simulink library "hapsrav_library"  (R2017a)
settings: Solver=VariableStepAuto  StartTime=0.0  StopTime=10.0  RelTol=1e-3
values from neighbouring files (symbols this model uses):
  absorb_h = 0:100:40000    [EnergySim.m]
  Adisk = pi * v.R_prop^2    [EnergySim.m]
  alpha_h = absorb_h    [EnergySim.m]
  aoa_data = zeros(n_cl, n)    [EnergySim.m]
  cl_bp = linspace(min_cl, max_cl,n_cl)    [EnergySim.m]
  D = [1       -.0065      288.15          0                   101325 ... (first row only)    [EnergySim.m]    (also in msn_params.m = sqrt((from_x - to_x)^2 + (from_y - to_y)^2); solar_vector.m = time.day + ut_time)
  d2r = pi / 180    (= 0.0174532925199)    [EnergySim.m]    (also in example1.m; example2.m; example3.m; example4.m)
  d_init = sqrt(dx*dx + dy*dy)    [EnergySim.m]    (also in msn_init.m)
  dchi0 = atan2(sin(dchi0), cos(dchi0))    [EnergySim.m]    (also in msn_init.m)
  dT = 0.5    [EnergySim.m]
  dT_fixed = 0.5    [EnergySim.m]
  dT_trig = 30    [EnergySim.m]
  earth_rho = 6378137.0    (= 6378137)    [EnergySim.m]
  fp = solarFP(p.orbit_rho, p.min_axis, p.orbit_dir, ic.x_ctr, ic.y_ctr, sun_az_0)    [EnergySim.m]    (also in load_fp.m = gid_tc(msn_idx).fp; solarFP.m = [1	6	2	nul eul 0	0	0	0	1	0)
  fp_coords = [x_entry y_entry]    [msn_params.m]
  fp_courses = [chi_adj nxt_chi dchi]    [msn_params.m]
  g = 9.80665    [EnergySim.m]
  Gsolar = 1367    [EnergySim.m]
  k = k+1    (= 5)    [EnergySim.m]
  K = D(:,2)    [EnergySim.m]
  lat_init = ic.lat_init_deg * obj.d2r    [EnergySim.m]
  M = time.month    [solar_vector.m]
  max_cl = max(cl_data(:))    [EnergySim.m]
  min_cl = min(cl_data(:))    [EnergySim.m]
  ND2 = load(fullfile(pwd,'nd2_data.mat'))    [EnergySim.m]    (also in nd2_data.mat = [0.0999999999999 0.200000000001 0.3 0.4 0.499999999998 0.700)
  next_init = fp(init_wp, 3)    [EnergySim.m]    (also in msn_init.m)
  pE_init = ic.pE_init    [EnergySim.m]
  pN_init = ic.pN_init    [EnergySim.m]
  r2d = 180 / pi    (= 57.2957795131)    [EnergySim.m]    (also in example1.m; example2.m; example3.m; example4.m)
  rho_SL = 1.225    [EnergySim.m]
  S = 110.4    [EnergySim.m]
  thr_lo_lim = 0.0    (= 0)    [EnergySim.m]
  time_init = struct('year', time.year, 'month', time.month,                  'day', time.day, 'hour', time.hour, 'min', time.min,                  'UTC', time.UTC)    [EnergySim.m]
  to_init = fp(init_wp, 1)    [EnergySim.m]    (also in msn_init.m)
  vgnd_init = sqrt(Vg)    [EnergySim.m]
  vtas_init = veas_init * sqrt(rho_sl/rho_alt)    [EnergySim.m]
  w_alt = 2.0 * w_alt    [EnergySim.m]
  w_xtrack = 2.0 * w_xtrack    [EnergySim.m]
undefined symbols (not defined in the file or in its folder): alpha, alpha_bp, alpha_circ, alt0_rate_init, alt_bp, alt_cmd_mode, alt_init, alt_lim_h, alt_lim_l, alt_rt_lim_periodic, cd_data, charge_eff, chi0_rate_init, chi_cmd_mode, chi_inf, chi_init, cl_data, discharge_eff, DiscIntNeverNeededParam, E_batt_max, E_init, Earth, enableFuzzyLogic, entry_init, epsln, epsln_circ, exit_init, f8_azimuth_offset, fig_eight_time, fp0, fp_coords0, fp_courses0, gamma_lim, hold_time, k_c, K_circ, lat_init_deg, lon_init_deg, max_alpha_bp, max_alt_bp, min_alpha_bp, min_alt_bp, min_axis, motor_eff, mppt_eff, num_motors, orb_dir_init, orb_len_init, orbit_dir, orbit_rho, P_acc, panel_eff, panel_vecs, phi_0, phi_lim, phi_lim_alt, phi_lim_alt_max, phi_lim_alt_min, phi_rt_lim, prop_eff_scale ... (+39)
libraries: simulink x59, hapsrav_library x9, fuzblock x3, atmospheric_library x1, aerolibtransform2 x1
(part 6 of 6)

== matlab function hapsrav_library/hapsrav_main/Kinematic 6DOF/Power Model/sun_position/sun_pos ==
  data: t1 input; sun_az output; t2 input; t3 input; t4 input; t5 input; t6 input; t7 input; l1 input; l2 input; l3 input; sun_zth output; jd output
function [sun_az, sun_zth, jd] = sun_position(t1, t2, t3, t4, t5, t6, t7, l1, l2, l3)
% sun = sun_position(time, location)
%
% This function compute the sun position (zenith and azimuth angle at the observer
% location) as a function of the observer local time and position. 
%
% It is an implementation of the algorithm presented by Reda et Andreas in:
%   Reda, I., Andreas, A. (2003) Solar position algorithm for solar
%   radiation application. National Renewable Energy Laboratory (NREL)
%   Technical report NREL/TP-560-34302. 
% This document is avalaible at www.osti.gov/bridge
%
% This algorithm is based on numerical approximation of the exact equations.
% The authors of the original paper state that this algorithm should be
% precise at +/- 0.0003 degrees. I have compared it to NOAA solar table
% (http://www.srrb.noaa.gov/highlights/sunrise/azel.html) and to USNO solar
% table (http://aa.usno.navy.mil/data/docs/AltAz.html) and found very good
% correspondance (up to the precision of those tables), except for large
% zenith angle, where the refraction by the atmosphere is significant 
% (difference of about 1 degree). Note that in this code the correction 
% for refraction in the atmosphere as been implemented for a temperature 
% of 10C (283 kelvins) and a pressure of 1010 mbar. See the subfunction 
% «sun_topocentric_zenith_angle_calculation» for a possible modification 
% to explicitely model the effect of temperature and pressure as describe
% in Reda & Andreas (2003). 
%
% Input parameters:
%   time: a structure that specify the time when the sun position is
%   calculated. 
%       time.year: year. Valid for [-2000, 6000]
%       time.month: month [1-12]
%       time.day: calendar day [1-31]
%       time.hour: local hour [0-23] (do not use DST)
%       time.min: minute [0-59]
%       time.sec: second [0-59]
%       time.UTC: offset hour from UTC. Local time = Greenwich time + time.UTC
%   This input can also be passed using the Matlab time format ('dd-mmm-yyyy HH:MM:SS'). 
%   In that case, the time has to be specified as UTC time (time.UTC = 0)
%
%   location: a structure that specify the location of the observer
%       location.latitude: latitude (in degrees, north of equator is
%       positive)
%       location.longitude: longitude (in degrees, positive for east of
%       Greenwich)
%       location.altitude: altitude above mean sea level (in meters) 
% 
% Output parameters
%   sun: a structure with the calculated sun position
%       sun.zenith = zenith angle in degrees (angle from the vertical)
%       sun.azimuth = azimuth angle in degrees, eastward from the north. 
% Only the sun zenith and azimuth angles are returned as output, but a lot
% of other parameters are calculated that could also extracted as output of
% this function. 
%
% Exemple of use
%
% location.longitude = -118.592421;
% location.latitude  =   34.181588;
% location.altitude  =  300.0;
% time.year = 2016;
% time.month = 10;
% time.day = 17;  %(do not use DST)
% time.hour = 9;
% time.min =  0;
% time.sec =  0;
% time.UTC = -8;
% 
% sun = sun_position(time, location);
%
% sun = 
% 
%      zenith: 57.8145
%      azimuth: 131.6647
%
% History
%   09/03/2004  Original creation by Vincent Roy (vincent.roy@drdc-rddc.gc.ca)
%   10/03/2004  Fixed a bug in julian_calculation subfunction (was
%               incorrect for year 1582 only), Vincent Roy
%   18/03/2004  Correction to the header (help display) only. No changes to
%               the code. (changed the «elevation» field in «location» structure
%               information to «altitude»), Vincent Roy
%   13/04/2004  Following a suggestion from Jody Klymak (jklymak@ucsd.edu),
%               allowed the 'time' input to be passed as a Matlab time string. 
%   22/08/2005  Following a bug report from Bruce Bowler
%               (bbowler@bigelow.org), modified the julian_calculation function. Bug
%               was 'MATLAB has allowed structure assignment  to a non-empty non-structure 
%               to overwrite the previous value.  This behavior will continue in this release, 
%               but will be an error in a  future version of MATLAB.  For advice on how to 
%               write code that  will both avoid this warning and work in future versions of 
%               MATLAB,  see R14SP2 Release Notes'. Script should now be
%               compliant with futher release of Matlab...

time.year = t1;
time.month = t2;
time.day = t3;
time.hour = t4;
time.min = t5;
time.sec = t6;
time.UTC = t7;

location.longitude = l1;
location.latitude = l2;
location.altitude = l3;

% 1. Calculate the Julian Day, and Century. Julian Ephemeris day, century
% and millenium are calculated using a mean delta_t of 33.184 seconds.  
julian = julian_calculation(time);
jd = mod(julian.day+13, 365.25);

% 2. Calculate the Earth heliocentric longitude, latitude, and radius
% vector (L, B, and R)
earth_heliocentric_position = earth_heliocentric_position_calculation(julian);

% 3. Calculate the geocentric longitude and latitude
sun_geocentric_position = sun_geocentric_position_calculation(earth_heliocentric_position);

% 4. Calculate the nutation in longitude and obliquity (in degrees). 
nutation = nutation_calculation(julian);

% 5. Calculate the true obliquity of the ecliptic (in degrees). 
true_obliquity = true_obliquity_calculation(julian, nutation);

% 6. Calculate the aberration correction (in degrees)
aberration_correction = abberation_correction_calculation(earth_heliocentric_position);

% 7. Calculate the apparent sun longitude in degrees)
apparent_sun_longitude = apparent_sun_longitude_calculation(sun_geocentric_position, nutation, aberration_correction);

% 8. Calculate the apparent sideral time at Greenwich (in degrees)
apparent_stime_at_greenwich = apparent_stime_at_greenwich_calculation(julian, nutation, true_obliquity);

% 9. Calculate the sun right ascension (in degrees)
sun_right_ascension = sun_right_ascension_calculation(apparent_sun_longitude, true_obliquity, sun_geocentric_position);

% 10. Calculate the geocentric sun declination (in degrees). Positive or
% negative if the sun is north or south of the celestial equator. 
sun_geocentric_declination = sun_geocentric_declination_calculation(apparent_sun_longitude, true_obliquity, sun_geocentric_position);

% 11. Calculate the observer local hour angle (in degrees, westward from south).
observer_local_hour = observer_local_hour_calculation(apparent_stime_at_greenwich, location, sun_right_ascension);

% 12. Calculate the topocentric sun position (right ascension, declination and
% right ascension parallax in degrees)
topocentric_sun_position = topocentric_sun_position_calculate(earth_heliocentric_position, location, observer_local_hour, sun_right_ascension, sun_geocentric_declination);

% 13. Calculate the topocentric local hour angle (in degrees)
topocentric_local_hour = topocentric_local_hour_calculate(observer_local_hour, topocentric_sun_position);

% 14. Calculate the topocentric zenith and azimuth angle (in degrees)
sun = sun_topocentric_zenith_angle_calculate(location, topocentric_sun_position, topocentric_local_hour);
sun_az = sun.azimuth;
sun_zth = sun.zenith;
end

%%%%%%%%%%%%%%%%%%%%%%%%%%%
% Subfunction definitions %
%%%%%%%%%%%%%%%%%%%%%%%%%%%

function julian = julian_calculation(t_input)
% This function compute the julian day and julian century from the local
% time and timezone information. Ephemeris are calculated with a delta_t=0
% seconds. 

% If time input is a Matlab time string, extract the information from
% this string and create the structure as defined in the main header of
% this script.
if ~isstruct(t_input)
    tt = datevec(t_input);
    time.UTC=0;
    time.year = tt(1);
    time.month = tt(2);
    time.day = tt(3);
    time.hour = tt(4);
    time.min = tt(5);
    time.sec = tt(6);
else
    time = t_input;
end

if(time.month == 1 || time.month == 2)
    Y = time.year - 1;
    M = time.month + 12;
else
    Y = time.year;
    M = time.month; 
end
ut_time = ((time.hour - time.UTC)/24) + (time.min/(60*24)) + (time.sec/(60*60*24)); % time of day in UT time. 
D = time.day + ut_time; % Day of month in decimal time, ex. 2sd day of month at 12:30:30UT, D=2.521180556

julian = struct('day',0,'ephemeris_day',0,'century',0,'ephemeris_century',0,'ephemeris_millenium',0);

% In 1582, the gregorian calendar was adopted
if(time.year == 1582)
    if(time.month == 10)
        if(time.day <= 4) % The Julian calendar ended on October 4, 1582
            B = 0;    
        elseif(time.day >= 15) % The Gregorian calendar started on October 15, 1582
            A = floor(Y/100);
            B = 2 - A + floor(A/4);    
        else
            disp('This date never existed!. Date automatically set to October 4, 1582');
            time.month = 10;
            time.day = 4; 
            B = 0;
        end
    elseif(time.month<10) % Julian calendar 
        B = 0;
    else % Gregorian calendar
        A = floor(Y/100);
        B = 2 - A + floor(A/4);
    end
    
elseif(time.year<1582) % Julian calendar
    B = 0;
else
    A = floor(Y/100); % Gregorian calendar
    B = 2 - A + floor(A/4);
end

julian.day = floor(365.25*(Y+4716)) + floor(30.6001*(M+1)) + D + B - 1524.5;

delta_t = 0; % 33.184;
julian.ephemeris_day = julian.day + (delta_t/86400);

julian.century = (julian.day - 2451545) / 36525; 

julian.ephemeris_century = (julian.ephemeris_day - 2451545) / 36525;

julian.ephemeris_millenium = julian.ephemeris_century / 10; 
end

function earth_heliocentric_position = earth_heliocentric_position_calculation(julian)
% This function compute the earth position relative to the sun, using
% tabulated values. 

% Tabulated values for the longitude calculation
% L terms  from the original code. 
 L0_terms = [175347046.0 0 0  
 3341656.0 4.6692568 6283.07585  
 34894.0 4.6261 12566.1517  
 3497.0 2.7441 5753.3849  
 3418.0 2.8289 3.5231  
 3136.0 3.6277 77713.7715  
 2676.0 4.4181 7860.4194  
 2343.0 6.1352 3930.2097  
 1324.0 0.7425 11506.7698  
 1273.0 2.0371 529.691  
 1199.0 1.1096 1577.3435  
 990 5.233 5884.927  
 902 2.045 26.298
 857 3.508 398.149  
 780 1.179 5223.694  
 753 2.533 5507.553  
 505 4.583 18849.228  
 492 4.205 775.523  
 357 2.92 0.067  
 317 5.849 11790.629  
 284 1.899 796.298  
 271 0.315 10977.079  
 243 0.345 5486.778  
 206 4.806 2544.314  
 205 1.869 5573.143  
 202 2.4458 6069.777  
 156 0.833 213.299  
 132 3.411 2942.463  
 126 1.083 20.775  
 115 0.645 0.98  
 103 0.636 4694.003  
 102 0.976 15720.839  
 102 4.267 7.114  
 99 6.21 2146.17  
 98 0.68 155.42  
 86 5.98 161000.69  
 85 1.3 6275.96  
 85 3.67 71430.7  
 80 1.81 17260.15  
 79 3.04 12036.46  
 71 1.76 5088.63  
 74 3.5 3154.69  
 74 4.68 801.82  
 70 0.83 9437.76  
 62 3.98 8827.39  
 61 1.82 7084.9  
 57 2.78 6286.6  
 56 4.39 14143.5  
 56 3.47 6279.55  
 52 0.19 12139.55  
 52 1.33 1748.02  
 51 0.28 5856.48  
 49 0.49 1194.45  
 41 5.37 8429.24  
 41 2.4 19651.05  
 39 6.17 10447.39  
 37 6.04 10213.29  
 37 2.57 1059.38  
 36 1.71 2352.87  
 36 1.78 6812.77  
 33 0.59 17789.85  
 30 0.44 83996.85  
 30 2.74 1349.87  
 25 3.16 4690.48];
 
L1_terms = [628331966747.0 0 0  
 206059.0 2.678235 6283.07585  
 4303.0 2.6351 12566.1517  
 425.0 1.59 3.523  
 119.0 5.796 26.298  
 109.0 2.966 1577.344  
 93 2.59 18849.23  
 72 1.14 529.69  
 68 1.87 398.15  
 67 4.41 5507.55  
 59 2.89 5223.69  
 56 2.17 155.42  
 45 0.4 796.3  
 36 0.47 775.52  
 29 2.65 7.11  
 21 5.34 0.98  
 19 1.85 5486.78  
 19 4.97 213.3  
 17 2.99 6275.96  
 16 0.03 2544.31  
 16 1.43 2146.17  
 15 1.21 10977.08
 12 2.83 1748.02  
 12 3.26 5088.63  
 12 5.27 1194.45  
 12 2.08 4694  
 11 0.77 553.57  
 10 1.3 3286.6  
 10 4.24 1349.87  
 9 2.7 242.73  
 9 5.64 951.72  
 8 5.3 2352.87  
 6 2.65 9437.76  
 6 4.67 4690.48]; 
  
L2_terms = [52919.0 0 0  
 8720.0 1.0721 6283.0758  
 309.0 0.867 12566.152  
 27 0.05 3.52  
 16 5.19 26.3  
 16 3.68 155.42  
 10 0.76 18849.23  
 9 2.06 77713.77  
 7 0.83 775.52  
 5 4.66 1577.34  
 4 1.03 7.11  
 4 3.44 5573.14  
 3 5.14 796.3  
 3 6.05 5507.55  
 3 1.19 242.73  
 3 6.12 529.69  
 3 0.31 398.15  
 3 2.28 553.57  
 2 4.38 5223.69  
 2 3.75 0.98];

L3_terms =[289.0 5.844 6283.076  
 35 0 0  
 17 5.49 12566.15  
 3 5.2 155.42  
 1 4.72 3.52  
 1 5.3 18849.23  
 1 5.97 242.73]; 
 
L4_terms = [114.0 3.142 0  
 8 4.13 6283.08  
 1 3.84 12566.15];

L5_terms = [1 3.14 0]; 

A0 = L0_terms(:,1);
B0 = L0_terms(:,2);
C0 = L0_terms(:,3);

A1 = L1_terms(:,1);
B1 = L1_terms(:,2);
C1 = L1_terms(:,3);

A2 = L2_terms(:,1);
B2 = L2_terms(:,2);
C2 = L2_terms(:,3);

A3 = L3_terms(:,1);
B3 = L3_terms(:,2);
C3 = L3_terms(:,3);

A4 = L4_terms(:,1);
B4 = L4_terms(:,2);
C4 = L4_terms(:,3);

A5 = L5_terms(:,1);
B5 = L5_terms(:,2);
C5 = L5_terms(:,3);

JME = julian.ephemeris_millenium;

% Compute the Earth Heliocentric longitude from the tabulated values. 
L0 = sum(A0 .* cos(B0 + (C0 * JME)));
L1 = sum(A1 .* cos(B1 + (C1 * JME)));
L2 = sum(A2 .* cos(B2 + (C2 * JME)));
L3 = sum(A3 .* cos(B3 + (C3 * JME)));
L4 = sum(A4 .* cos(B4 + (C4 * JME)));
L5 = A5 .* cos(B5 + (C5 * JME));


earth_heliocentric_position = struct('longitude',0,'latitude',0,'radius',0);

earth_heliocentric_position.longitude = (L0 + (L1 * JME) + (L2 * JME^2) + (L3 * JME^3) + (L4 * JME^4) + (L5 * JME^5)) / 1e8; 
% Convert the longitude to degrees. 
earth_heliocentric_position.longitude = earth_heliocentric_position.longitude * 180/pi;
% Limit the range to [0,360[;
earth_heliocentric_position.longitude = set_to_range(earth_heliocentric_position.longitude, 0, 360);

% Tabulated values for the earth heliocentric latitude. 
% B terms  from the original code. 
 B0_terms = [280.0 3.199 84334.662  
 102.0 5.422 5507.553  
 80 3.88 5223.69  
 44 3.7 2352.87  
 32 4 1577.34]; 
  
B1_terms = [9 3.9 5507.55  
 6 1.73 5223.69]; 

A0 = B0_terms(:,1);
B0 = B0_terms(:,2);
C0 = B0_terms(:,3);

A1 = B1_terms(:,1);
B1 = B1_terms(:,2);
C1 = B1_terms(:,3);

L0 = sum(A0 .* cos(B0 + (C0 * JME)));
L1 = sum(A1 .* cos(B1 + (C1 * JME)));

earth_heliocentric_position.latitude = (L0 + (L1 * JME)) / 1e8; 
% Convert the latitude to degrees. 
earth_heliocentric_position.latitude = earth_heliocentric_position.latitude * 180/pi;
% Limit the range to [0,360];
earth_heliocentric_position.latitude = set_to_range(earth_heliocentric_position.latitude, 0, 360);

% Tabulated values for radius vector. 
% R terms from the original code
R0_terms = [ 100013989.0 0 0  
 1670700.0 3.0984635 6283.07585  
 13956.0 3.05525 12566.1517   
 3084.0 5.1985 77713.7715  
 1628.0 1.1739 5753.3849  
 1576.0 2.8469 7860.4194  
 925.0 5.453 11506.77  
 542.0 4.564 3930.21  
 472.0 3.661 5884.927  
 346.0 0.964 5507.553  
 329.0 5.9 5223.694  
 307.0 0.299 5573.143  
 243.0 4.273 11790.629  
 212.0 5.847 1577.344  
 186.0 5.022 10977.079  
 175.0 3.012 18849.228  
 110.0 5.055 5486.778  
 98 0.89 6069.78  
 86 5.69 15720.84  
 86 1.27 161000.69  
 85 0.27 17260.15  
 63 0.92 529.69  
 57 2.01 83996.85  
 56 5.24 71430.7  
 49 3.25 2544.31  
 47 2.58 775.52  
 45 5.54 9437.76  
 43 6.01 6275.96  
 39 5.36 4694  
 38 2.39 8827.39  
 37 0.83 19651.05  
 37 4.9 12139.55  
 36 1.67 12036.46  
 35 1.84 2942.46  
 33 0.24 7084.9  
 32 0.18 5088.63  
 32 1.78 398.15  
 28 1.21 6286.6  
 28 1.9 6279.55  
 26 4.59 10447.39];
   
R1_terms = [ 103019.0 1.10749 6283.07585  
 1721.0 1.0644 12566.1517  
 702.0 3.142 0  
 32 1.02 18849.23  
 31 2.84 5507.55  
 25 1.32 5223.69  
 18 1.42 1577.34  
 10 5.91 10977.08  
 9 1.42 6275.96  
 9 0.27 5486.78];
  
R2_terms = [4359.0 5.7846 6283.0758  
 124.0 5.579 12566.152  
 12 3.14 0  
 9 3.63 77713.77  
 6 1.87 5573.14  
 3 5.47 18849];
 
R3_terms = [145.0 4.273 6283.076  
 7 3.92 12566.15];

R4_terms = [4 2.56 6283.08];


A0 = R0_terms(:,1);
B0 = R0_terms(:,2);
C0 = R0_terms(:,3);

A1 = R1_terms(:,1);
B1 = R1_terms(:,2);
C1 = R1_terms(:,3);

A2 = R2_terms(:,1);
B2 = R2_terms(:,2);
C2 = R2_terms(:,3);

A3 = R3_terms(:,1);
B3 = R3_terms(:,2);
C3 = R3_terms(:,3);

A4 = R4_terms(:,1);
B4 = R4_terms(:,2);
C4 = R4_terms(:,3);

% Compute the Earth heliocentric radius vector
L0 = sum(A0 .* cos(B0 + (C0 * JME)));
L1 = sum(A1 .* cos(B1 + (C1 * JME)));
L2 = sum(A2 .* cos(B2 + (C2 * JME)));
L3 = sum(A3 .* cos(B3 + (C3 * JME)));
L4 = A4 .* cos(B4 + (C4 * JME));

% Units are in AU
earth_heliocentric_position.radius = (L0 + (L1 * JME) + (L2 * JME^2) + (L3 * JME^3) + (L4 * JME^4)) / 1e8; 

end

function sun_geocentric_position = sun_geocentric_position_calculation(earth_heliocentric_position)
% This function compute the sun position relative to the earth. 
sun_geocentric_position = struct('longitude',0,'latitude',0);

sun_geocentric_position.longitude = earth_heliocentric_position.longitude + 180;
% Limit the range to [0,360];
sun_geocentric_position.longitude = set_to_range(sun_geocentric_position.longitude, 0, 360);

sun_geocentric_position.latitude = -earth_heliocentric_position.latitude;
% Limit the range to [0,360]
sun_geocentric_position.latitude = set_to_range(sun_geocentric_position.latitude, 0, 360);
end

function nutation = nutation_calculation(julian)
% This function compute the nutation in longtitude and in obliquity, in
% degrees. 

% All Xi are in degrees. 
JCE = julian.ephemeris_century;

% 1. Mean elongation of the moon from the sun 
p = [(1/189474) -0.0019142 445267.11148 297.85036];
% X0 = polyval(p, JCE);
X0 = p(1) * JCE^3 + p(2) * JCE^2 + p(3) * JCE + p(4); % This is faster than polyval...

% 2. Mean anomaly of the sun (earth)
p = [-(1/300000) -0.0001603 35999.05034 357.52772];
% X1 = polyval(p, JCE);
X1 = p(1) * JCE^3 + p(2) * JCE^2 + p(3) * JCE + p(4); 

% 3. Mean anomaly of the moon
p = [(1/56250) 0.0086972 477198.867398 134.96298];
% X2 = polyval(p, JCE);
X2 = p(1) * JCE^3 + p(2) * JCE^2 + p(3) * JCE + p(4); 

% 4. Moon argument of latitude
p = [(1/327270) -0.0036825 483202.017538 93.27191];
% X3 = polyval(p, JCE);
X3 = p(1) * JCE^3 + p(2) * JCE^2 + p(3) * JCE + p(4); 

% 5. Longitude of the ascending node of the moon's mean orbit on the
% ecliptic, measured from the mean equinox of the date
p = [(1/450000) 0.0020708 -1934.136261 125.04452];
% X4 = polyval(p, JCE);
X4 = p(1) * JCE^3 + p(2) * JCE^2 + p(3) * JCE + p(4); 

% Y tabulated terms from the original code
Y_terms =  [0 0 0 0 1  
 -2 0 0 2 2  
 0 0 0 2 2  
 0 0 0 0 2  
 0 1 0 0 0  
 0 0 1 0 0  
 -2 1 0 2 2  
 0 0 0 2 1  
 0 0 1 2 2  
 -2 -1 0 2 2  
 -2 0 1 0 0  
 -2 0 0 2 1  
 0 0 -1 2 2  
 2 0 0 0 0  
 0 0 1 0 1  
 2 0 -1 2 2  
 0 0 -1 0 1  
 0 0 1 2 1  
 -2 0 2 0 0  
 0 0 -2 2 1  
 2 0 0 2 2  
 0 0 2 2 2  
 0 0 2 0 0  
 -2 0 1 2 2  
 0 0 0 2 0  
 -2 0 0 2 0  
 0 0 -1 2 1  
 0 2 0 0 0  
 2 0 -1 0 1  
 -2 2 0 2 2  
 0 1 0 0 1  
 -2 0 1 0 1  
 0 -1 0 0 1  
 0 0 2 -2 0  
 2 0 -1 2 1  
 2 0 1 2 2  
 0 1 0 2 2  
 -2 1 1 0 0  
 0 -1 0 2 2  
 2 0 0 2 1  
 2 0 1 0 0  
 -2 0 2 2 2  
 -2 0 1 2 1  
 2 0 -2 0 1  
 2 0 0 0 1  
 0 -1 1 0 0  
 -2 -1 0 2 1  
 -2 0 0 0 1  
 0 0 2 2 1  
 -2 0 2 0 1  
 -2 1 0 2 1  
 0 0 1 -2 0  
 -1 0 1 0 0  
 -2 1 0 0 0  
 1 0 0 0 0  
 0 0 1 2 0  
 0 0 -2 2 2  
 -1 -1 1 0 0  
 0 1 1 0 0  
 0 -1 1 2 2  
 2 -1 -1 2 2  
 0 0 3 2 2  
 2 -1 0 2 2];

nutation_terms = [ -171996 -174.2 92025 8.9  
 -13187 -1.6 5736 -3.1  
 -2274 -0.2 977 -0.5  
 2062 0.2 -895 0.5  
 1426 -3.4 54 -0.1  
 712 0.1 -7 0  
 -517 1.2 224 -0.6  
 -386 -0.4 200 0  
 -301 0 129 -0.1  
 217 -0.5 -95 0.3  
 -158 0 0 0  
 129 0.1 -70 0  
 123 0 -53 0  
 63 0 0 0  
 63 0.1 -33 0  
 -59 0 26 0  
 -58 -0.1 32 0  
 -51 0 27 0  
 48 0 0 0  
 46 0 -24 0  
 -38 0 16 0  
 -31 0 13 0  
 29 0 0 0  
 29 0 -12 0  
 26 0 0 0  
 -22 0 0 0  
 21 0 -10 0  
 17 -0.1 0 0  
 16 0 -8 0  
 -16 0.1 7 0  
 -15 0 9 0  
 -13 0 7 0  
 -12 0 6 0  
 11 0 0 0  
 -10 0 5 0  
 -8 0 3 0  
 7 0 -3 0  
 -7 0 0 0  
 -7 0 3 0  
 -7 0 3 0  
 6 0 0 0  
 6 0 -3 0  
 6 0 -3 0  
 -6 0 3 0  
 -6 0 3 0  
 5 0 0 0  
 -5 0 3 0  
 -5 0 3 0  
 -5 0 3 0  
 4 0 0 0  
 4 0 0 0  
 4 0 0 0  
 -4 0 0 0  
 -4 0 0 0  
 -4 0 0 0  
 3 0 0 0  
 -3 0 0 0  
 -3 0 0 0  
 -3 0 0 0  
 -3 0 0 0  
 -3 0 0 0  
 -3 0 0 0  
 -3 0 0 0];

% Using the tabulated values, compute the delta_longitude and
% delta_obliquity. 
Xi = [X0
    X1
    X2
    X3
    X4];

tabulated_argument = (Y_terms * Xi) * pi/180;

delta_longitude = ((nutation_terms(:,1) + (nutation_terms(:,2) * JCE))) .* sin(tabulated_argument);
delta_obliquity = ((nutation_terms(:,3) + (nutation_terms(:,4) * JCE))) .* cos(tabulated_argument);

% Nutation in longitude
nutation.longitude = sum(delta_longitude) / 36000000;

% Nutation in obliquity
nutation.obliquity = sum(delta_obliquity) / 36000000;
end

function true_obliquity = true_obliquity_calculation(julian, nutation)
% This function compute the true obliquity of the ecliptic. 


p = [2.45 5.79 27.87 7.12 -39.05 -249.67 -51.38 1999.25 -1.55 -4680.93 84381.448];
% mean_obliquity = polyval(p, julian.ephemeris_millenium/10);

U = julian.ephemeris_millenium/10;
mean_obliquity = p(1)*U^10 + p(2)*U^9 + p(3)*U^8 + p(4)*U^7 + p(5)*U^6 + p(6)*U^5 + p(7)*U^4 + p(8)*U^3 + p(9)*U^2 + p(10)*U + p(11);


true_obliquity = (mean_obliquity/3600) + nutation.obliquity;
end

function aberration_correction = abberation_correction_calculation(earth_heliocentric_position)
% This function compute the aberration_correction, as a function of the
% earth-sun distance. 

aberration_correction = -20.4898/(3600*earth_heliocentric_position.radius);
end

function apparent_sun_longitude = apparent_sun_longitude_calculation(sun_geocentric_position, nutation, aberration_correction)
% This function compute the sun apparent longitude

apparent_sun_longitude = sun_geocentric_position.longitude + nutation.longitude + aberration_correction;
end

function apparent_stime_at_greenwich = apparent_stime_at_greenwich_calculation(julian, nutation, true_obliquity)
% This function compute the apparent sideral time at Greenwich. 

JD = julian.day;
JC = julian.century;

% Mean sideral time, in degrees
mean_stime = 280.46061837 + (360.98564736629*(JD-2451545)) + (0.000387933*JC^2) - (JC^3/38710000);

% Limit the range to [0-360];
mean_stime = set_to_range(mean_stime, 0, 360);

apparent_stime_at_greenwich = mean_stime + (nutation.longitude * cos(true_obliquity * pi/180));
end

function sun_right_ascension = sun_right_ascension_calculation(apparent_sun_longitude, true_obliquity, sun_geocentric_position)
% This function compute the sun right ascension. 

argument_numerator = (sin(apparent_sun_longitude * pi/180) * cos(true_obliquity * pi/180)) - ...
    (tan(sun_geocentric_position.latitude * pi/180) * sin(true_obliquity * pi/180));
argument_denominator = cos(apparent_sun_longitude * pi/180);

sun_right_ascension = atan2(argument_numerator, argument_denominator) * 180/pi;
% Limit the range to [0,360];
sun_right_ascension = set_to_range(sun_right_ascension, 0, 360);
end

function sun_geocentric_declination = sun_geocentric_declination_calculation(apparent_sun_longitude, true_obliquity, sun_geocentric_position)

argument = (sin(sun_geocentric_position.latitude * pi/180) * cos(true_obliquity * pi/180)) + ...
    (cos(sun_geocentric_position.latitude * pi/180) * sin(true_obliquity * pi/180) * sin(apparent_sun_longitude * pi/180));

sun_geocentric_declination = asin(argument) * 180/pi;
end

function observer_local_hour = observer_local_hour_calculation(apparent_stime_at_greenwich, location, sun_right_ascension)

observer_local_hour = apparent_stime_at_greenwich + location.longitude - sun_right_ascension;
% Set the range to [0-360]
observer_local_hour = set_to_range(observer_local_hour, 0, 360);

end

function topocentric_sun_position = topocentric_sun_position_calculate(earth_heliocentric_position, location, observer_local_hour, sun_right_ascension, sun_geocentric_declination)
% This function compute the sun position (right ascension and declination)
% with respect to the observer local position at the Earth surface. 

% Equatorial horizontal parallax of the sun in degrees
eq_horizontal_parallax = 8.794 / (3600 * earth_heliocentric_position.radius);

% Term u, used in the following calculations (in radians)
u = atan(0.99664719 * tan(location.latitude * pi/180));

% Term x, used in the following calculations
x = cos(u) + ((location.altitude/6378140) * cos(location.latitude * pi/180));

% Term y, used in the following calculations
y = (0.99664719 * sin(u)) + ((location.altitude/6378140) * sin(location.latitude * pi/180));

% Parallax in the sun right ascension (in radians)
nominator = -x * sin(eq_horizontal_parallax * pi/180) * sin(observer_local_hour * pi/180);
denominator = cos(sun_geocentric_declination * pi/180) - (x * sin(eq_horizontal_parallax * pi/180) * cos(observer_local_hour * pi/180));
sun_right_ascension_parallax = atan2(nominator, denominator);
% Conversion to degrees. 
topocentric_sun_position.right_ascension_parallax = sun_right_ascension_parallax * 180/pi;

% Topocentric sun right ascension (in degrees)
topocentric_sun_position.right_ascension = sun_right_ascension + (sun_right_ascension_parallax * 180/pi);

% Topocentric sun declination (in degrees)
nominator = (sin(sun_geocentric_declination * pi/180) - (y*sin(eq_horizontal_parallax * pi/180))) * cos(sun_right_ascension_parallax);
denominator = cos(sun_geocentric_declination * pi/180) - (x*sin(eq_horizontal_parallax * pi/180)) * cos(observer_local_hour * pi/180);
topocentric_sun_position.declination = atan2(nominator, denominator) * 180/pi;
end

function topocentric_local_hour = topocentric_local_hour_calculate(observer_local_hour, topocentric_sun_position)
% This function compute the topocentric local jour angle in degrees

topocentric_local_hour = observer_local_hour - topocentric_sun_position.right_ascension_parallax;
end

function sun = sun_topocentric_zenith_angle_calculate(location, topocentric_sun_position, topocentric_local_hour)
% This function compute the sun zenith angle, taking into account the
% atmospheric refraction. A default temperature of 283K and a
% default pressure of 1010 mbar are used. 

% Topocentric elevation, without atmospheric refraction
argument = (sin(location.latitude * pi/180) * sin(topocentric_sun_position.declination * pi/180)) + ...
    (cos(location.latitude * pi/180) * cos(topocentric_sun_position.declination * pi/180) * cos(topocentric_local_hour * pi/180));
true_elevation = asin(argument) * 180/pi;

% Atmospheric refraction correction (in degrees)
argument = true_elevation + (10.3/(true_elevation + 5.11));
refraction_corr = 1.02 / (60 * tan(argument * pi/180));

% For exact pressure and temperature correction, use this, 
% with P the pressure in mbar amd T the temperature in Kelvins:
% refraction_corr = (P/1010) * (283/T) * 1.02 / (60 * tan(argument * pi/180));

% Apparent elevation
if(true_elevation > -5)
    apparent_elevation = true_elevation + refraction_corr;
else
    apparent_elevation = true_elevation;
end

sun.zenith = 90 - apparent_elevation;


% Topocentric azimuth angle. The +180 conversion is to pass from astronomer
% notation (westward from south) to navigation notation (eastward from
% north);
nominator = sin(topocentric_local_hour * pi/180);
denominator = (cos(topocentric_local_hour * pi/180) * sin(location.latitude * pi/180)) - ...
    (tan(topocentric_sun_position.declination * pi/180) * cos(location.latitude * pi/180));
sun.azimuth = (atan2(nominator, denominator) * 180/pi) + 180;
% Set the range to [0-360]
sun.azimuth = set_to_range(sun.azimuth, 0, 360);
end

function var = set_to_range(var, min_interval, max_interval)
% if(var>0)
%     var = var - max_interval * floor(var/max_interval);
% else
%     var = var - max_interval * ceil(var/max_interval);
% end
% 
% if(var<min_interval)
%     var = var + max_interval;
% end

var = var - max_interval * floor(var/max_interval);

if(var<min_interval)
    var = var + max_interval;
end
end

== matlab function hapsrav_library/hapsrav_main/Kinematic 6DOF/Power Model/sun_position/time_update ==
  data: time_init input; t_new output; sim_secs input
function t_new = fcn(time_init, sim_secs)
coder.extrinsic('datetime');
coder.extrinsic('datevec');

time_now = time_init + sim_secs;
t_new = zeros(6,1);

    if ~coder.target('MATLAB')
        coder.cinclude('<stdio.h>');
        coder.cinclude('<time.h>');
        coder.cinclude('date_vec.h');

        t_new(1) = coder.ceval('get_year',time_now);
        t_new(2) = coder.ceval('get_month',time_now);
        t_new(3) = coder.ceval('get_day',time_now);
        t_new(4) = coder.ceval('get_hour',time_now);
        t_new(5) = coder.ceval('get_min',time_now);
        t_new(6) = coder.ceval('get_sec',time_now);
    else
        dt_now = datetime(time_now,'ConvertFrom','posixtime');
        t_new_tmp = datevec(dt_now);
        t_new = t_new_tmp';
    end
end

== matlab function hapsrav_library/Cmd - Parametric/Chi Cmd/Circular Vector Fields/MATLAB Function1 ==
  data: av_x input; av_y input; d output; x_c input; y_c input; orbit_dir input; g output; beta output; r_c input; chi_d output; k_c input
function [d,g,beta,chi_d] = relPosn(av_x, av_y, x_c, y_c, orbit_dir, r_c, k_c)

x = av_x;
y = av_y;
% x_c = to_x
% y_c = to_y;

dx = x - x_c;
dy = y - y_c;

d = sqrt(dx * dx + dy * dy);
g = atan2(dy, dx);       % correct as dy, dx

ang_y = k_c * (d - r_c);
ang_x = r_c;

if (orbit_dir)
    % CCW
    chi_d = g - pi/2 - atan(ang_y/ ang_x);
else
    % CW
    chi_d = g + pi/2 + atan(ang_y/ ang_x);
end

chi_d = wrap2pi(chi_d);

% Compute beta
d_err = d - r_c;
k_r = k_c / r_c;
beta = k_r / (1 + (k_r * d_err)^2);


end

function wrpd = wrap2pi(angl)

% Wrap to +/- pi
if (angl > pi)
    wrpd = -pi + (angl - pi);
elseif (angl < -pi)
    wrpd = 2 * pi + angl;
else
    wrpd = angl;
end

end

== matlab function hapsrav_library/hapsrav_main/Kinematic 6DOF/Selectable Modes/Trajectory_Optimization/Roll/roll_angle/Limited Integration ==
  data: u input; y0 output; T input; uplim input; lolim input; x0 input; x1 output
function [y0,x1] = lim_integr(u, T, uplim, lolim, x0)

K = 1.0;

y0   = x0 + K * T/2 * u;
y0 = max(min(y0, uplim), lolim);
x1   = y0 + K * T/2 * u;

end

== matlab function hapsrav_library/Cmd - Parametric/Chi Cmd/Circular Vector Fields/MATLAB Function3 ==
  data: chi input; chi_cmd output; d input; g input; chi_d input; beta input; Vg input; alpha input; e input; K input
function chi_cmd = chiCmdCirc(chi, d, g, chi_d, beta, Vg, alpha, e, K)

chi_err = wrap2pi(chi - chi_d);
angl = chi - g;
angl = wrap2pi(angl);

chi_cmd = chi + Vg * sin(angl) / alpha / d;
chi_cmd = chi_cmd - beta * Vg * cos(angl) / alpha;

satVal = sat_val(chi_err, e);
chi_cmd = chi_cmd - K * satVal / alpha;
chi_cmd = wrap2pi(chi_cmd);

end

function satVal = sat_val(u,epsln)

x = u / epsln;

if (abs(x) <= 1)
    satVal = x;
else
    satVal = sign(x);
end

end

function wrpd = wrap2pi(angl)

% Wrap to +/- pi
if (angl > pi)
    wrpd = -pi + (angl - pi);
elseif (angl < -pi)
    wrpd = 2 * pi + angl;
else
    wrpd = angl;
end

end

== matlab function hapsrav_library/hapsrav_main/Kinematic 6DOF/Selectable Modes/Waypoint_Navigation/Course/MATLAB Function2 ==
  data: ref input; circ_err output; posn input
function circ_err  = circErr(ref, posn)
% Assumes that both angles are limited to the range +/-pi
% Replace this function with a summing junction
% to see why it's needed.  Go thru a sign change
% in the error.

s1 = sign(ref);
s2 = sign(posn);

err = ref - posn;

if (s1 > s2),
    if (abs(err) > pi),
        err = err - 2*pi;
    end
elseif (s2 > s1),
    if (abs(err) > pi),
        err = 2*pi + err;
    end
end

% When error is exactly +/-pi, want to add option to continue
% turning along same direction
circ_err = err;

end

== matlab function hapsrav_library/hapsrav_main/Kinematic 6DOF/Selectable Modes/Waypoint_Navigation/Course/chi_dot/Limited Integration ==
  data: u input; y0 output; T input; lim input; x0 input; x1 output
function [y0,x1] = lim_integr(u, T, lim, x0)

K = 1.0;

y0   = x0 + K * T/2 * u;

y0 = max(min(y0, lim), -lim);

x1   = y0 + K * T/2 * u;

end

== stateflow chart hapsrav_library/Cmd - Parametric/Chi Cmd/Flight Plan/Mission Director/Fly Away Detection ==
  state Not_Fly_Away
    %
    entry:
    fly_away_flg = false;
  state Counting
    %
    entry:
    fly_away_ctr = 500;
    during:
    fly_away_ctr = fly_away_ctr - 1;
  state Fly_Away
    %
    entry:
    fly_away_flg = true;
  (default) -> Not_Fly_Away
  Fly_Away -> Not_Fly_Away : [d2n >= turn_rad]
  Counting -> Not_Fly_Away [order 1] : [~retreating]
  Not_Fly_Away -> Counting : [(d2n < turn_rad) && ...
      | retreating]
  Counting -> Fly_Away [order 2] : [fly_away_ctr == 0]
  data: d2n input; retreating input; turn_rad input; fly_away_flg output boolean; fly_away_ctr local

== matlab function hapsrav_library/Cmd - Parametric/Chi Cmd/Flight Plan/Mission Director/MATLAB Function ==
  data: wp_upd input; wp_upd_old input; wp_to output; wp_entry input; wp_curr input; wp_next input
function wp_to  = fcn(wp_upd, wp_upd_old, wp_entry, wp_curr, wp_next)

if (wp_upd == 0)
    wp_to = wp_entry;
elseif (wp_upd ~= wp_upd_old)
    wp_to = wp_next;
else
    wp_to = wp_curr;
end

end

== stateflow chart hapsrav_library/Cmd - Parametric/Chi Cmd/Flight Plan/Mission Director/Mission Director ==
  state Not_Entry_Mode
    state Orbit_Holding_Mode
      state Pattern_Hold_Entry
        %
        entry:
        orbit_timer = 50 * orbit_time;
        sweeping = false;
        state_flg = -2;
      state Pattern_Hold
        state Entry
          %
          entry:
          nav_mode = 3;
          state_flg = -3;
        state Sweep_Exit_Mode
          entry:
          sweeping = true;
          state_flg = 5;
        state Timer_Exit_Mode
          entry:
          state_flg = 4;
          during:
          orbit_timer = orbit_timer - 1;
        (default) -> Not_Entry_Mode.Orbit_Holding_Mode.Pattern_Hold.Entry
        Not_Entry_Mode.Orbit_Holding_Mode.Pattern_Hold.Entry -> Sweep_Exit_Mode [order 2] : [sweep_flg]
        Not_Entry_Mode.Orbit_Holding_Mode.Pattern_Hold.Entry -> Timer_Exit_Mode [order 1] : [~sweep_flg]
      state Fly_Over_Mode	% 2
        %
        entry:
        if (nav_mode ~= 0)
        nav_mode = 2;
        end
        delay_timer = 50 * 4;
        state_flg = 3;
        during:
        delay_timer = delay_timer -1;
      (default) -> Pattern_Hold_Entry
      Pattern_Hold_Entry -> Pattern_Hold [order 1] : [fly_over_flg ~= 2]
      Pattern_Hold_Entry -> Fly_Over_Mode	% 2 [order 2] : [fly_over_flg == 2]
      Fly_Over_Mode	% 2 -> Pattern_Hold : [delay_timer == 0]
    state Entry
      entry:
      state_flg = -1;
    state Path_Following_Mode		% 2
      %
      entry:
      nav_mode = 2;
      state_flg = 2;
    state Turning_Mode 	% 0
      %
      entry:
      nav_mode = 1;
      state_flg = 1;
    (default) -> Not_Entry_Mode.Entry
    Not_Entry_Mode.Entry -> Orbit_Holding_Mode [order 1] : [orbit_flg]
    Not_Entry_Mode.Entry -> Turning_Mode 	% 0 [order 2] : [~orbit_flg]
        | {wp_upd = wp_upd + 1;}
    Orbit_Holding_Mode -> (junction 183) [order 2] : [~sweep_flg && sweeping]
    Orbit_Holding_Mode -> (junction 183) [order 1] : [orbit_timer == 0]
    Path_Following_Mode		% 2 -> Orbit_Holding_Mode [order 2] : [orbit_flg && ...
        | (d2n < prox_dist)]
    (junction 183) -> Path_Following_Mode		% 2 : {wp_upd = wp_upd + 1;}
    Path_Following_Mode		% 2 -> Turning_Mode 	% 0 [order 1] : [~orbit_flg && ...
        | ((d2n < prox_dist) || fly_away_flg)]
        | {wp_upd = wp_upd + 1;}
    Turning_Mode 	% 0 -> Path_Following_Mode		% 2 : [d2n >= prox_dist]
  state Entry_Mode	% 1
    %
    entry:
    wp_upd = 0;
    msn_rst = 1;
    nav_mode = 0;
    state_flg = 0;
    %
    during:
    msn_rst = 0;
  (default) -> Entry_Mode	% 1
  Entry_Mode	% 1 -> Not_Entry_Mode : [d2n < prox_dist]
  Not_Entry_Mode -> Entry_Mode	% 1 : % 2
      | [Ovrd]
  data: Ovrd input; d2n input; wp_upd output; nav_mode output; prox_dist input; orbit_time input; msn_rst output; orbit_timer local; delay_timer local; orbit_flg input; fly_over_flg input; fly_away_flg input; sweep_flg input; sweeping local boolean; state_flg output

== matlab function hapsrav_library/Cmd - Parametric/Chi Cmd/Flight Plan/Mission Director/Nav Leg/Flight Plan/Realtime FP/MATLAB Function ==
  data: fp output; fp_courses output; fp_coords output; maj_axis input; min_axis input; orbit_dir input; x_ctr input; y_ctr input; az input
function [fp, fp_courses, fp_coords] = update_fp(maj_axis, min_axis, orbit_dir, x_ctr, y_ctr, az)

nc = x_ctr;
ec = y_ctr;

rho = min_axis;
drho = maj_axis - min_axis;

nu_ctr = nc + drho * cos(az);
eu_ctr = ec + drho * sin(az);

nur = nu_ctr - rho * sin(az);
eur = eu_ctr + rho * cos(az);
nul = nu_ctr + rho * sin(az);
eul = eu_ctr - rho * cos(az);

nl_ctr = nc - drho * cos(az);
el_ctr = ec - drho * sin(az);

nlr = nl_ctr - rho * sin(az);
elr = el_ctr + rho * cos(az);
nll = nl_ctr + rho * sin(az);
ell = el_ctr - rho * cos(az);

% orbit direction: 1 - CCW, 0 - CW
if (orbit_dir)  % CCW
    fp = [1	6	2	nur eur 0	0	0	0	1	0;
        2	1	3   nu_ctr eu_ctr 1	min_axis	1	180	3	5;
        3	2	4   nul eul 0	0	0	0	1	0;
        4	3	5   nll ell 0	0	0	0	1	0;
        5	4	6   nl_ctr el_ctr 1	min_axis	1	180	3	5;
        6	5	1   nlr elr 0	0	0	0	1	0];
else    % CW
    fp = [1	6	2	nul eul 0	0	0	0	1	0;
        2	1	3	nu_ctr eu_ctr 1	min_axis	0	180	3	5;
        3	2	4	nur eur 0	0	0	0	1	0;
        4	3	5	nlr elr 0	0	0	0	1	0;
        5	4	6	nl_ctr el_ctr 1	min_axis	0	180	3	5;
        6	5	1	nll ell 0	0	0	0	1	0];
end

[fp_courses, fp_coords] = msn_params(fp);

end

function [fp_courses, fp_coords] = msn_params(fp)
%
num_wp = 6;

chi_nom    = zeros(num_wp,1);	% course of this leg (to, from)
chi_adj    = zeros(num_wp,1);   % course of next leg (next, to)
nxt_chi    = zeros(num_wp,1);   % course of next leg (next, to)
dchi       = zeros(num_wp,1);   % change in course

x_entry = zeros(num_wp,1);
y_entry = zeros(num_wp,1);

for i = 1:num_wp
    
    % Compute chi, next_chi, delta_chi
    to_wp = fp(i, 1);
    from_wp = fp(i, 2);
    
    to_x = fp(to_wp, 4);
    to_y = fp(to_wp, 5);
    from_x = fp(from_wp, 4);
    from_y = fp(from_wp, 5);
    
    dy = to_y - from_y;
    dx = to_x - from_x;
    chi_nom(i) = atan2(dy,dx);
    
    % Compute entry point for intercept patternholds
    % whenever intercept and orbit are both defined
    if (fp(i,10) == 3)
%         % Circle parameters
%         %rho = fp(to_wp, 7);
%         %D = sqrt((from_x - to_x)^2 + (from_y - to_y)^2);
%         %gamma = pi/2 - acos(rho / D);
%         gamma = pi/2;
%         %De = sqrt(D*D - rho*rho);
%         De = 0.0;
%         
%         if (fp(to_wp,8) > 0)    % CCW
%             chi_adj(i) = chi_nom(i) + gamma;
%         else                    % CW
%             chi_adj(i) = chi_nom(i) - gamma;
%         end
%         
%         %y_entry(i) = from_y + De * sin(chi_adj(i));
%         %x_entry(i) = from_x + De * cos(chi_adj(i));
%         
%         y_entry(i) = from_y;
%         x_entry(i) = from_x;

        % Circle parameters
        rho = fp(to_wp, 7);
        D = sqrt((from_x - to_x)^2 + (from_y - to_y)^2);
        % problem when rho > D
        if (rho > D)
            gamma = pi/2;
            De = 0.0;
        else 
            gamma = pi/2 - acos(rho / D);
            De = sqrt(D*D - rho*rho);
        end
        
        if (fp(to_wp,8) > 0)    % CCW
            chi_adj(i) = chi_nom(i) + gamma;
        else                    % CW
            chi_adj(i) = chi_nom(i) - gamma;
        end
        
        y_entry(i) = from_y + De * sin(chi_adj(i));
        x_entry(i) = from_x + De * cos(chi_adj(i));
    else
        chi_adj(i) = chi_nom(i);
        x_entry(i) = to_x;
        y_entry(i) = to_y;
    end
end

for i = 1:num_wp
    % Compute next_chi, delta_chi
	next_wp = fp(i, 3);
    nxt_chi(i) = chi_adj(next_wp);
end

% Compute dchi using the actual entry points
%nxt_chi = [chi_adj(2:end);chi_adj(1)];

delta_crs = nxt_chi - chi_adj;
dchi = atan2(sin(delta_crs),cos(delta_crs));

fp_courses = [chi_adj nxt_chi dchi];
fp_coords = [x_entry y_entry];

end

== matlab function hapsrav_library/Cmd - Parametric/Chi Cmd/Flight Plan/Mission Director/Proximity Distance/MATLAB Function ==
  data: ang input; ang2pi output
function ang2pi = fcn(ang)
%   
%   Wrap to [0, 2pi]
%
    if (ang < 0)
        ang2pi = ang + 2 * pi;
    else
        ang2pi = ang;
    end
end
